simulink model "Main_Data_Flow"  (R2023a)
settings: Solver=FixedStepAuto  StartTime=0.0  StopTime=10.0  FixedStep=1e-3  RelTol=1e-3  EnableMultiTasking=on
undefined symbols (not defined in the file): D0, D1, D10, D11, D12, D13, D14, D15, D2, D3, D4, D5, D6, D7, D8, D9, PTA0, PTA1, PTA2, PTB23, PTB9, PTC16, PTC17, PTC2, PTC3, PTC4, PTD0, PTD1, PTD2, PTD3, PTE24, PTE25
libraries: frdmk64flib x33
settings Model: ExtModeTrigDuration=5  Creator=sadeg  LastModifiedBy=sadeg
settings OptimizationCC: EnhancedBackFolding=on  PassReuseOutputArgsAs=Individual arguments  ZeroExternalMemoryAtStartup=off  ZeroInternalMemoryAtStartup=off  MaxStackSize=64  OptimizeBlockOrder=speed  DifferentSizesBufferReuse=on  OptimizationCustomize=off  EfficientTunableParamExpr=on
settings DebuggingCC: ParameterTunabilityLossMsg=error
settings HardwareCC: ProdBitPerPointer=32  ProdBitPerSizeT=32  ProdBitPerPtrDiffT=32  ProdLargestAtomicInteger=Long  ProdLargestAtomicFloat=Double  ProdWordSize=32  ProdHWDeviceType=ARM Compatible->ARM Cortex  UseEmbeddedCoderFeatures=off
settings SFSimCC: MATLABDynamicMemAlloc=off
settings RTWCC: Description=Embedded Coder  SystemTargetFile=ert.tlc  HardwareBoard=NXP FRDM-K64F  TLCOptions="-aInlineSetEventsForThisBaseRateFcn=TLC_FALSE -aSuppressMultiTaskScheduler=TLC_FALSE  -aRateBasedStepFcn=0"  TemplateMakefile=ert_default_tmf  Toolchain=GNU Tools for ARM Embedded Processors
settings CodeAppCC: ForceParamTrailComments=on  IgnoreCustomStorageClasses=off  OperatorAnnotations=on  SimulinkDataObjDesc=on  SFDataObjDesc=on  InsertBlockDesc=on
settings ERTTargetCC: SupportNonInlinedSFcns=on  ExtModeTransport=4  ExtModeMexFile=sendToCommService

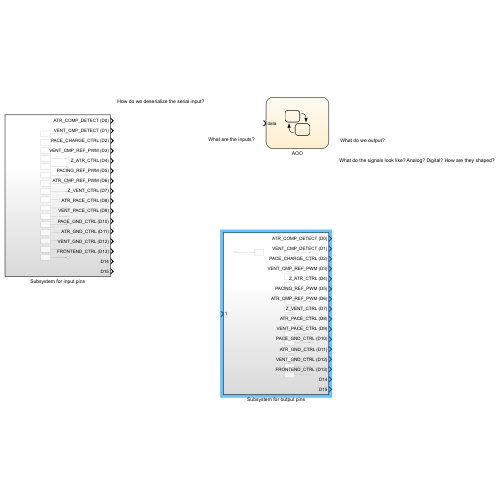
[thumbnail: Simulink's stored preview of the top-level diagram]
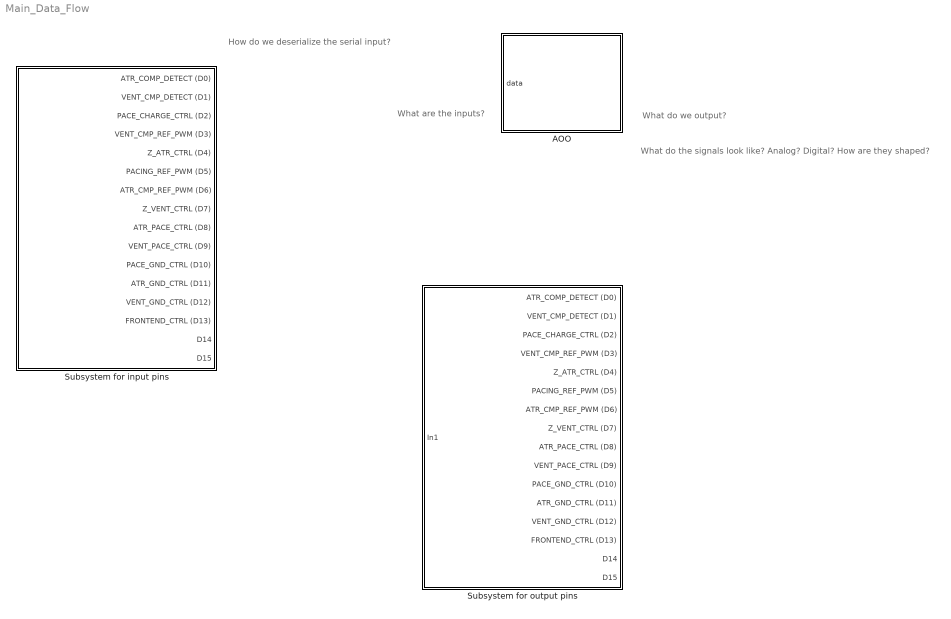
== system Main_Data_Flow ==
  note: What do the signals look like? Analog? Digital? How are they shaped?
  note: What do we output?
  note: How do we deserialize the serial input?
  note: What are the inputs?
  AOO : Stateflow chart  TreatAsAtomicUnit=on
  Subsystem for input pins : Subsystem
  Subsystem for output pins : Subsystem

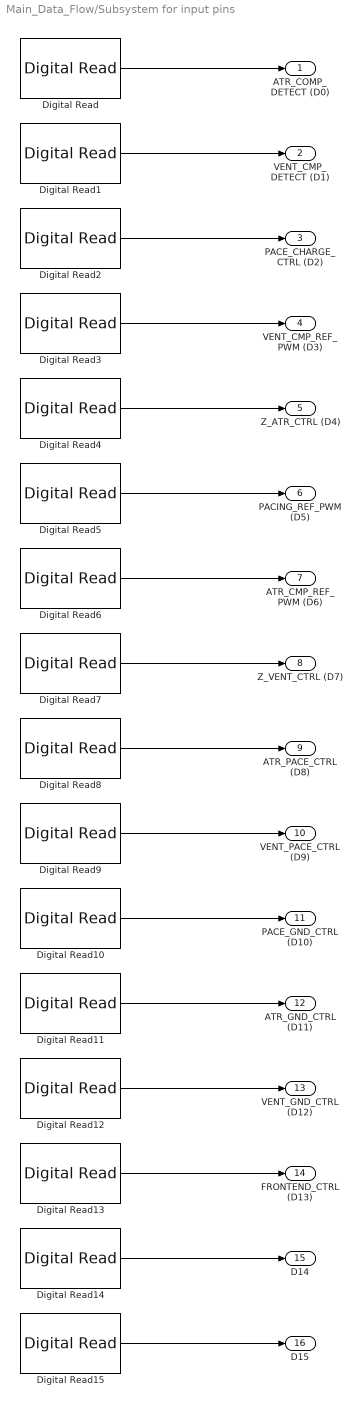
== system Main_Data_Flow/Subsystem for input pins ==
  Digital Read : frdmk64flib/Digital Read  Whichpin=PTC16 (D0)  SampleTime=-1
  Digital Read1 : frdmk64flib/Digital Read  Whichpin=PTC17 (D1)  SampleTime=-1
  Digital Read10 : frdmk64flib/Digital Read  Whichpin=PTD0 (D10)  SampleTime=-1
  Digital Read11 : frdmk64flib/Digital Read  Whichpin=PTD2 (D11)  SampleTime=-1
  Digital Read12 : frdmk64flib/Digital Read  Whichpin=PTD3 (D12)  SampleTime=-1
  Digital Read13 : frdmk64flib/Digital Read  Whichpin=PTD1 (D13)  SampleTime=-1
  Digital Read14 : frdmk64flib/Digital Read  Whichpin=PTE25 (D14)  SampleTime=-1
  Digital Read15 : frdmk64flib/Digital Read  Whichpin=PTE24 (D15)  SampleTime=-1
  Digital Read2 : frdmk64flib/Digital Read  Whichpin=PTB9 (D2)  SampleTime=-1
  Digital Read3 : frdmk64flib/Digital Read  Whichpin=PTA1 (D3)  SampleTime=-1
  Digital Read4 : frdmk64flib/Digital Read  Whichpin=PTB23 (D4)  SampleTime=-1
  Digital Read5 : frdmk64flib/Digital Read  Whichpin=PTA2 (D5)  SampleTime=-1
  Digital Read6 : frdmk64flib/Digital Read  Whichpin=PTC2 (D6)  SampleTime=-1
  Digital Read7 : frdmk64flib/Digital Read  Whichpin=PTC3 (D7)  SampleTime=-1
  Digital Read8 : frdmk64flib/Digital Read  Whichpin=PTA0 (D8)  SampleTime=-1
  Digital Read9 : frdmk64flib/Digital Read  Whichpin=PTC4 (D9)  SampleTime=-1
  ATR_COMP_DETECT (D0) : Outport
  VENT_CMP_DETECT (D1) : Outport  Port=2
  PACE_CHARGE_CTRL (D2) : Outport  Port=3
  VENT_CMP_REF_PWM (D3) : Outport  Port=4
  Z_ATR_CTRL (D4) : Outport  Port=5
  PACING_REF_PWM (D5) : Outport  Port=6
  ATR_CMP_REF_PWM (D6) : Outport  Port=7
  Z_VENT_CTRL (D7) : Outport  Port=8
  ATR_PACE_CTRL (D8) : Outport  Port=9
  VENT_PACE_CTRL (D9) : Outport  Port=10
  PACE_GND_CTRL (D10) : Outport  Port=11
  ATR_GND_CTRL (D11) : Outport  Port=12
  VENT_GND_CTRL (D12) : Outport  Port=13
  FRONTEND_CTRL (D13) : Outport  Port=14
  D14 : Outport  Port=15
  D15 : Outport  Port=16
  wires:
  Digital Read/1 -> ATR_COMP_DETECT (D0)/1
  Digital Read1/1 -> VENT_CMP_DETECT (D1)/1
  Digital Read2/1 -> PACE_CHARGE_CTRL (D2)/1
  Digital Read3/1 -> VENT_CMP_REF_PWM (D3)/1
  Digital Read4/1 -> Z_ATR_CTRL (D4)/1
  Digital Read5/1 -> PACING_REF_PWM (D5)/1
  Digital Read6/1 -> ATR_CMP_REF_PWM (D6)/1
  Digital Read7/1 -> Z_VENT_CTRL (D7)/1
  Digital Read8/1 -> ATR_PACE_CTRL (D8)/1
  Digital Read10/1 -> PACE_GND_CTRL (D10)/1
  Digital Read14/1 -> D14/1
  Digital Read9/1 -> VENT_PACE_CTRL (D9)/1
  Digital Read11/1 -> ATR_GND_CTRL (D11)/1
  Digital Read12/1 -> VENT_GND_CTRL (D12)/1
  Digital Read13/1 -> FRONTEND_CTRL (D13)/1
  Digital Read15/1 -> D15/1

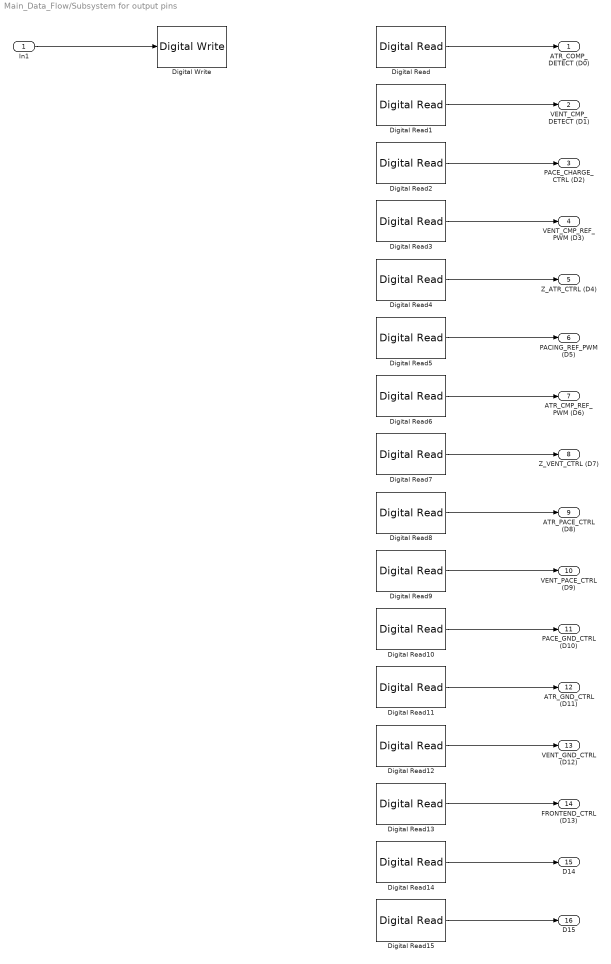
== system Main_Data_Flow/Subsystem for output pins ==
  In1 : Inport
  Digital Read : frdmk64flib/Digital Read  Whichpin=PTC16 (D0)  SampleTime=-1
  Digital Read1 : frdmk64flib/Digital Read  Whichpin=PTC17 (D1)  SampleTime=-1
  Digital Read10 : frdmk64flib/Digital Read  Whichpin=PTD0 (D10)  SampleTime=-1
  Digital Read11 : frdmk64flib/Digital Read  Whichpin=PTD2 (D11)  SampleTime=-1
  Digital Read12 : frdmk64flib/Digital Read  Whichpin=PTD3 (D12)  SampleTime=-1
  Digital Read13 : frdmk64flib/Digital Read  Whichpin=PTD1 (D13)  SampleTime=-1
  Digital Read14 : frdmk64flib/Digital Read  Whichpin=PTE25 (D14)  SampleTime=-1
  Digital Read15 : frdmk64flib/Digital Read  Whichpin=PTE24 (D15)  SampleTime=-1
  Digital Read2 : frdmk64flib/Digital Read  Whichpin=PTB9 (D2)  SampleTime=-1
  Digital Read3 : frdmk64flib/Digital Read  Whichpin=PTA1 (D3)  SampleTime=-1
  Digital Read4 : frdmk64flib/Digital Read  Whichpin=PTB23 (D4)  SampleTime=-1
  Digital Read5 : frdmk64flib/Digital Read  Whichpin=PTA2 (D5)  SampleTime=-1
  Digital Read6 : frdmk64flib/Digital Read  Whichpin=PTC2 (D6)  SampleTime=-1
  Digital Read7 : frdmk64flib/Digital Read  Whichpin=PTC3 (D7)  SampleTime=-1
  Digital Read8 : frdmk64flib/Digital Read  Whichpin=PTA0 (D8)  SampleTime=-1
  Digital Read9 : frdmk64flib/Digital Read  Whichpin=PTC4 (D9)  SampleTime=-1
  Digital Write : frdmk64flib/Digital Write  Whichpin=PTC16 (D0)
  ATR_COMP_DETECT (D0) : Outport
  VENT_CMP_DETECT (D1) : Outport  Port=2
  PACE_CHARGE_CTRL (D2) : Outport  Port=3
  VENT_CMP_REF_PWM (D3) : Outport  Port=4
  Z_ATR_CTRL (D4) : Outport  Port=5
  PACING_REF_PWM (D5) : Outport  Port=6
  ATR_CMP_REF_PWM (D6) : Outport  Port=7
  Z_VENT_CTRL (D7) : Outport  Port=8
  ATR_PACE_CTRL (D8) : Outport  Port=9
  VENT_PACE_CTRL (D9) : Outport  Port=10
  PACE_GND_CTRL (D10) : Outport  Port=11
  ATR_GND_CTRL (D11) : Outport  Port=12
  VENT_GND_CTRL (D12) : Outport  Port=13
  FRONTEND_CTRL (D13) : Outport  Port=14
  D14 : Outport  Port=15
  D15 : Outport  Port=16
  wires:
  Digital Read/1 -> ATR_COMP_DETECT (D0)/1
  Digital Read1/1 -> VENT_CMP_DETECT (D1)/1
  Digital Read2/1 -> PACE_CHARGE_CTRL (D2)/1
  Digital Read3/1 -> VENT_CMP_REF_PWM (D3)/1
  Digital Read4/1 -> Z_ATR_CTRL (D4)/1
  Digital Read5/1 -> PACING_REF_PWM (D5)/1
  Digital Read6/1 -> ATR_CMP_REF_PWM (D6)/1
  Digital Read7/1 -> Z_VENT_CTRL (D7)/1
  Digital Read8/1 -> ATR_PACE_CTRL (D8)/1
  Digital Read10/1 -> PACE_GND_CTRL (D10)/1
  Digital Read14/1 -> D14/1
  Digital Read9/1 -> VENT_PACE_CTRL (D9)/1
  Digital Read11/1 -> ATR_GND_CTRL (D11)/1
  Digital Read12/1 -> VENT_GND_CTRL (D12)/1
  Digital Read13/1 -> FRONTEND_CTRL (D13)/1
  Digital Read15/1 -> D15/1
  In1/1 -> Digital Write/1

== stateflow chart Main_Data_Flow/AOO ==
  data: data input
